simulink model "system_origin"  (R2015b)
settings: Solver=VariableStepAuto  StartTime=0.0  StopTime=10  RelTol=1e-3
settings Model: Creator=kazuhiro  LastModifiedBy=kazuhiro

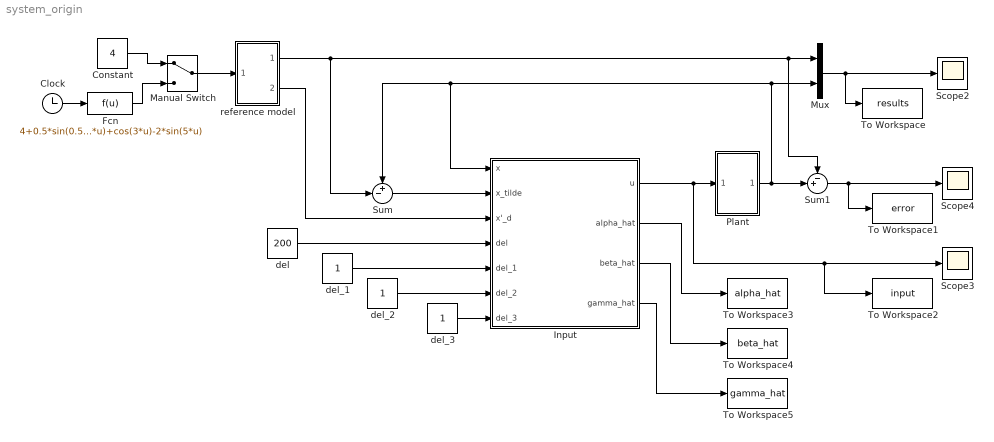
== system system_origin ==
  Clock : Clock
  Constant : Constant  Value=4
  Fcn : Fcn  Expr=4+0.5*sin(0.5*u)+cos(3*u)-2*sin(5*u)
  Input : Subsystem
  Manual Switch : ManualSwitch
  Mux : Mux  Inputs=2
  Plant : Subsystem
  Scope2 : Scope
  Scope3 : Scope
  Scope4 : Scope
  Sum : Sum  Inputs=+-|
  Sum1 : Sum  Inputs=-+|
  To Workspace : ToWorkspace  VariableName=results  SampleTime=-1
  To Workspace1 : ToWorkspace  VariableName=error  SampleTime=-1
  To Workspace2 : ToWorkspace  VariableName=input  SampleTime=-1
  To Workspace3 : ToWorkspace  VariableName=alpha_hat  SampleTime=-1
  To Workspace4 : ToWorkspace  VariableName=beta_hat  SampleTime=-1
  To Workspace5 : ToWorkspace  VariableName=gamma_hat  SampleTime=-1
  del : Constant  Value=200
  del_1 : Constant
  del_2 : Constant
  del_3 : Constant
  reference model : Subsystem
  wires:
  Input/1(u) -> To Workspace2/1, Scope3/1, Plant/1(u(t))
  Manual Switch/1 -> reference model/1(r_d)
  Constant/1 -> Manual Switch/1
  Clock/1 -> Fcn/1
  Fcn/1 -> Manual Switch/2
  reference model/2(x'_d) -> Input/3(x'_d)
  del/1 -> Input/4("del ")
  del_2/1 -> Input/6(del_2)
  del_3/1 -> Input/7(del_3)
  Plant/1(x(t)) -> Sum/1, Input/1(x), Mux/2, Sum1/2
  reference model/1(x_d) -> Sum/2, Sum1/1, Mux/1
  del_1/1 -> Input/5(del_1)
  Sum/1 -> Input/2(x_tilde)
  Mux/1 -> To Workspace/1, Scope2/1
  Sum1/1 -> Scope4/1, To Workspace1/1
  Input/2(alpha_hat) -> To Workspace3/1
  Input/3(beta_hat) -> To Workspace4/1
  Input/4(gamma_hat) -> To Workspace5/1

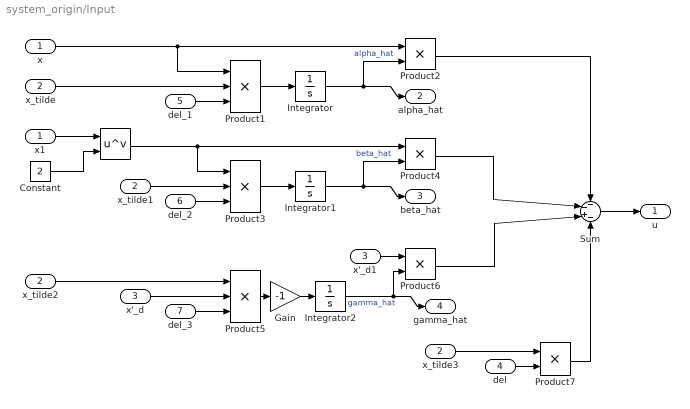
== system system_origin/Input ==
  x : Inport
  x_tilde : Inport  Port=2
  x'_d : Inport  Port=3
  "del " : Inport  Port=4
  del_1 : Inport  Port=5
  del_2 : Inport  Port=6
  del_3 : Inport  Port=7
  " " : Math  Operator=pow  SaturateOnIntegerOverflow=on
  Constant : Constant  Value=2
  Gain : Gain  Gain=-1
  Integrator : Integrator
  Integrator1 : Integrator
  Integrator2 : Integrator
  Product1 : Product  Inputs=3
  Product{2,4,6..7} (4 alike) : Product
  Product3 : Product  Inputs=3
  Product5 : Product  Inputs=3
  Sum : Sum  Inputs=--+-
  x'_d1 : InportShadow  Port=3
  x1 : InportShadow
  x_tilde1 : InportShadow  Port=2
  x_tilde2 : InportShadow  Port=2
  x_tilde3 : InportShadow  Port=2
  u : Outport
  alpha_hat : Outport  Port=2
  beta_hat : Outport  Port=3
  gamma_hat : Outport  Port=4
  wires:
  Product2/1 -> Sum/1
  x_tilde/1 -> Product1/2
  x/1 -> Product2/1, Product1/1
  Integrator/1 -> alpha_hat/1, Product2/2  "alpha_hat"
  Product1/1 -> Integrator/1
  del_1/1 -> Product1/3
  Product4/1 -> Sum/2
  x_tilde1/1 -> Product3/2
  " "/1 -> Product3/1, Product4/1
  Integrator1/1 -> Product4/2, beta_hat/1  "beta_hat"
  Product3/1 -> Integrator1/1
  del_2/1 -> Product3/3
  x1/1 -> " "/1
  Constant/1 -> " "/2
  Product6/1 -> Sum/3
  x'_d/1 -> Product5/2
  Integrator2/1 -> gamma_hat/1, Product6/2  "gamma_hat"
  del_3/1 -> Product5/3
  Product5/1 -> Gain/1
  Gain/1 -> Integrator2/1
  x'_d1/1 -> Product6/1
  "del "/1 -> Product7/2
  x_tilde2/1 -> Product5/1
  x_tilde3/1 -> Product7/1
  Product7/1 -> Sum/4
  Sum/1 -> u/1

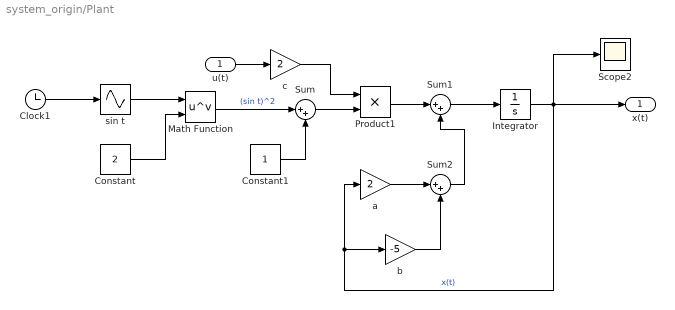
== system system_origin/Plant ==
  u(t) : Inport
  Clock1 : Clock
  Constant : Constant  Value=2
  Constant1 : Constant
  Integrator : Integrator
  Math Function : Math  Operator=pow  SaturateOnIntegerOverflow=on
  Product1 : Product
  Scope2 : Scope
  Sum : Sum  Inputs=|++
  Sum1 : Sum  Inputs=|++
  Sum2 : Sum  Inputs=|++
  a : Gain  Gain=2
  b : Gain  Gain=-5
  "c " : Gain  Gain=2
  sin t : Sin  TimeSource=Use external signal  SampleTime=0
  x(t) : Outport
  wires:
  sin t/1 -> Math Function/1
  a/1 -> Sum2/1
  "c "/1 -> Product1/1
  Math Function/1 -> Sum/1  "(sin t)^2"
  b/1 -> Sum2/2
  u(t)/1 -> "c "/1
  Sum/1 -> Product1/2
  Sum1/1 -> Integrator/1
  Constant1/1 -> Sum/2
  Product1/1 -> Sum1/1
  Sum2/1 -> Sum1/2
  Integrator/1 -> a/1, b/1, x(t)/1, Scope2/1  "x(t)"
  Clock1/1 -> sin t/1
  Constant/1 -> Math Function/2

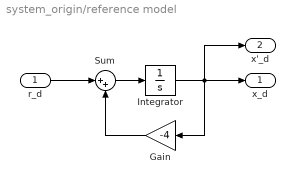
== system system_origin/reference model ==
  r_d : Inport
  Gain : Gain  Gain=-4
  Integrator : Integrator
  Sum : Sum  Inputs=|++
  x_d : Outport
  x'_d : Outport  Port=2
  wires:
  Gain/1 -> Sum/2
  r_d/1 -> Sum/1
  Integrator/1 -> x_d/1, Gain/1, x'_d/1
  Sum/1 -> Integrator/1
